simulink model "RealAndSimulatedPlantBlock2019"  (R2019b)
settings: Solver=FixedStepAuto  StartTime=0.0  StopTime=60  FixedStep=0.001  RelTol=1e-3
values from neighbouring files (symbols this model uses):
  A = [0 0 0 0 1 -7.46314951586 0 9.2203186001 0 -3.6743536316 0 36.5167723042 ... (16 elements, 4x4)]    [PlantParams.mat]
  B = [0 5.59662878796 0 -6.91433293703]    [PlantParams.mat]
  c = 0.2    [PlantParams.mat]    (also in params.m = 0.1)
  dtheta1 = 41.8879020479    [PlantParams.mat]    (also in params.m)
  g = 9.81    [PlantParams.mat]    (also in params.m)
  Id = 0.0148    [PlantParams.mat]    (also in params.m)
  ID = 0.0148142940058    [PlantParams.mat]
  J1 = 0.13138281053    [PlantParams.mat]    (also in params.m = 0.1314)
  JC = 0.0268600431258    [PlantParams.mat]
  JD = 0.0273039035837    [PlantParams.mat]
  Jz_bar = 0.0130765    [PlantParams.mat]    (also in params.m = 0.0131)
  lcg = 0.269778481013    [PlantParams.mat]    (also in params.m = 0.2698)
  m = 0.158    [PlantParams.mat]    (also in params.m)
  rh = 0.37    [PlantParams.mat]    (also in params.m)
undefined symbols (not defined in the file or in its folder): C, D, X, Y, Z
libraries: sm_lib x20, nesl_utility x5, simulink x1
(part 2 of 2)

== matlab function RealAndSimulatedPlantBlock2019/Plant/Non-linear Simulation Plant/Subsystem/MATLAB Function ==
  data: theta_ddot_1 output; theta_2 input; theta_3 input; theta_4 input; theta_dot_1 input; theta_dot_2 input; theta_dot_3 input; theta_dot_4 input; T_1 input; T_2 input; theta_ddot_2 output; theta_ddot_3 output; theta_ddot_4 output
function [theta_ddot_1, theta_ddot_2, theta_ddot_3, theta_ddot_4] = ...
    fcn(theta_2, theta_3, theta_4, theta_dot_1,...
        theta_dot_2, theta_dot_3, theta_dot_4, T_1, T_2)
g = 9.81;
theta_ddot_1 = -(1958372730237732701804682603107415175787744873616217473024000*T_1 - 366215700554455999080225274065048781396920318332014769625*theta_dot_1 + 237406127304858667686861471985309025571272801769849956875*theta_dot_1*cos(theta_2)^2 + 128809573249597331393363802079739755825647516562164812750*theta_dot_1*cos(theta_3)^2 + 217352965440431972313920503751859592659321613927317504000*theta_dot_1*cos(theta_4)^2 + 52359703185237910572295885124678117792802251079355468750*theta_dot_1*sin(theta_3)^2 + 3427789003866943481470413557670984804612355776241773576192*theta_dot_3*sin(theta_2) - 1269551482913682770914967984322586964671242880089545768960000*T_1*cos(theta_2)^2 - 688821247324049930889714618784828211116501993526671704064000*T_1*cos(theta_3)^2 - 1162315323210866213387287415560227994624885237945177473024000*T_1*cos(theta_4)^2 - 279998412755282956590263894637395024770552498749440000000000*T_1*sin(theta_3)^2 - 53471220207419015071532913264009106990133399900755204620000*theta_dot_2*theta_dot_3*cos(theta_2) + 753492488642099239087836691412794808278935743167945768960000*T_1*cos(theta_2)^2*cos(theta_4)^2 + 408822834568766974299450724147433186345949494777231704064000*T_1*cos(theta_3)^2*cos(theta_4)^2 - 140903095376072551492852586796797954626476348444508160000*theta_dot_1*cos(theta_2)^2*cos(theta_4)^2 - 76449870064359420821067916955061638032845265482809344000*theta_dot_1*cos(theta_3)^2*cos(theta_4)^2 + 9403754461680578526877673084778282939987100019066108660000*theta_dot_3^2*sin(2*theta_3)*sin(theta_2) + 34663711284057858017777567094452541110159199862622987300000*theta_dot_2*theta_dot_3*cos(theta_2)^3 - 516058994271583531827131292909792156392307136921600000000000*T_2*sin(theta_2)*sin(theta_3) + 6089496132404685675560149256335547445429224215674880000000*theta_dot_2*sin(theta_2)*sin(theta_3) + 688821247324049930889714618784828211116501993526671704064000*T_1*cos(theta_2)^2*cos(theta_3) - 128809573249597331393363802079739755825647516562164812750*theta_dot_1*cos(theta_2)^2*cos(theta_3) - 2034429719333667945537159066814545982353126506553453576192*theta_dot_3*cos(theta_4)^2*sin(theta_2) + 34663711284057858017777567094452541110159199862622987300000*theta_dot_1*theta_dot_2*cos(theta_2)*sin(theta_2) + 76449870064359420821067916955061638032845265482809344000*theta_dot_1*cos(theta_2)^2*cos(theta_3)*cos(theta_4)^2 - 9403754461680578526877673084778282939987100019066108660000*theta_dot_3^2*cos(theta_2)^2*sin(theta_2)*sin(theta_3) - 7045212511554242352783209429865101928420942356832031250000*theta_dot_3^2*sin(2*theta_2)*sin(theta_2)*sin(theta_3) + 18807508923361157053755346169556565879974200038132217320000*theta_dot_2*theta_dot_3*cos(theta_2)*cos(theta_3)^2 + 31735745518842579422338363526619723554514196982000517120000*theta_dot_2*theta_dot_3*cos(theta_2)*cos(theta_4)^2 - 18807508923361157053755346169556565879974200038132217320000*theta_dot_2*theta_dot_3*cos(theta_2)^3*cos(theta_3) + 7645049665467950943628130877659179578777318205090625000000*theta_dot_2*theta_dot_3*cos(theta_2)*sin(theta_3)^2 + 34663711284057858017777567094452541110159199862622987300000*theta_dot_2*theta_dot_3*sin(2*theta_2)*sin(theta_2) + 7077726405892498128003306834840222747846164275527680000*theta_dot_4*cos(theta_4)*sin(theta_2)*sin(theta_3) - 5581229628946603055063607645948693150598440916520796160000*theta_dot_3^2*sin(2*theta_3)*cos(theta_4)^2*sin(theta_2) - 20573286260949373312211148234722337253317315148958924800000*theta_dot_2*theta_dot_3*cos(theta_2)^3*cos(theta_4)^2 - 7645049665467950943628130877659179578777318205090625000000*theta_dot_3^2*cos(theta_3)*sin(theta_2)*sin(theta_3) + 8138895413405711776328644403303559546502173933174784000000*theta_dot_4^2*sin(theta_2)*sin(theta_3)*sin(theta_4) - 408822834568766974299450724147433186345949494777231704064000*T_1*cos(theta_2)^2*cos(theta_3)*cos(theta_4)^2 + 7645049665467950943628130877659179578777318205090625000000*theta_dot_3^2*cos(theta_2)*cos(theta_3)*sin(theta_2)^2*sin(theta_3) - 20573286260949373312211148234722337253317315148958924800000*theta_dot_1*theta_dot_2*cos(theta_2)*cos(theta_4)^2*sin(theta_2) - 37615017846722314107510692339113131759948400076264434640000*theta_dot_2*theta_dot_3*cos(theta_2)*cos(theta_3)*sin(theta_2)^2 - 30168808805116773270614095383506449462694275224436736000000*g*cos(theta_4)*sin(theta_2)*sin(theta_3)*sin(theta_4) + 5581229628946603055063607645948693150598440916520796160000*theta_dot_3^2*cos(theta_2)^2*cos(theta_4)^2*sin(theta_2)*sin(theta_3) - 11162459257893206110127215291897386301196881833041592320000*theta_dot_2*theta_dot_3*cos(theta_2)*cos(theta_3)^2*cos(theta_4)^2 + 11162459257893206110127215291897386301196881833041592320000*theta_dot_2*theta_dot_3*cos(theta_2)^3*cos(theta_3)*cos(theta_4)^2 - 20573286260949373312211148234722337253317315148958924800000*theta_dot_2*theta_dot_3*sin(2*theta_2)*cos(theta_4)^2*sin(theta_2) - 14090425023108484705566418859730203856841884713664062500000*theta_dot_1*theta_dot_3*cos(theta_2)*sin(theta_2)*sin(theta_3) + 22324918515786412220254430583794772602393763666083184640000*theta_dot_2*theta_dot_3*cos(theta_2)*cos(theta_3)*cos(theta_4)^2*sin(theta_2)^2)/(10734426842075824580000*(3229209327524243103578455495267868185*cos(theta_2)^2 + 1752073883408586258584044588908630554*cos(theta_3)^2 + 2956445275163430863787903017879076864*cos(theta_4)^2 + 3229209327524243103578455495267868185*sin(theta_2)^2 + 712199149329667464909054858375156250*sin(theta_3)^2 - 1752073883408586258584044588908630554*cos(theta_2)^2*cos(theta_3) - 1916570541084512070112913287345602560*cos(theta_2)^2*cos(theta_4)^2 - 1039874734078918793674989730533474304*cos(theta_3)^2*cos(theta_4)^2 - 1916570541084512070112913287345602560*cos(theta_4)^2*sin(theta_2)^2 + 1039874734078918793674989730533474304*cos(theta_2)^2*cos(theta_3)*cos(theta_4)^2 - 4981283210932829362162500084176498739));
theta_ddot_2 = (8799655665284731983770664469744582656000*theta_dot_2 - 7457335309563332189636156330292019200000000*T_2 - 5704540165669006975595484450903818240000*theta_dot_2*cos(theta_2)^2 - 3095115499615725008175180018840764416000*theta_dot_2*cos(theta_3)^2 - 110475157775578382071318015937187337500000*theta_dot_3^2*cos(theta_3) - 5704540165669006975595484450903818240000*theta_dot_2*sin(theta_2)^2 + 117611499500950702795799230524118007808000*theta_dot_4^2*sin(theta_4) + 38857585587426656885438033072948525000000*theta_dot_3^2*cos(theta_3)^3 - 101807182141934847986128970358377296875000*theta_dot_3^2*sin(2*theta_2) + 10227702573538355420671664494284374016*theta_dot_4*cos(theta_4) + 7082043939798692815316089873618698240000*theta_dot_3*sin(theta_3) + 4834356072600853369148715636359168000000000*T_2*cos(theta_2)^2 + 2622979236962478820487440693932851200000000*T_2*cos(theta_3)^2 + 4834356072600853369148715636359168000000000*T_2*sin(theta_2)^2 - 203614364283869695972257940716754593750000*theta_dot_1*theta_dot_3*cos(theta_2) + 71617572188151725185879982864238812500000*theta_dot_3^2*cos(theta_2)^2*cos(theta_3) + 71617572188151725185879982864238812500000*theta_dot_3^2*cos(theta_3)*sin(theta_2)^2 - 76243838210006208698186681479929528320000*theta_dot_4^2*cos(theta_2)^2*sin(theta_4) - 41367661290944494097612549044188479488000*theta_dot_4^2*cos(theta_3)^2*sin(theta_4) + 19428792793713328442719016536474262500000*theta_dot_3^2*sin(2*theta_3)*sin(theta_3) - 76243838210006208698186681479929528320000*theta_dot_4^2*sin(theta_2)^2*sin(theta_4) + 131996792095717970786377957852515781250000*theta_dot_1*theta_dot_3*cos(theta_2)^3 + 2622979236962478820487440693932851200000000*T_1*sin(theta_2)*sin(theta_3) - 435955822197072399806129699068871442432000*g*cos(theta_4)*sin(theta_4) - 38857585587426656885438033072948525000000*theta_dot_3^2*cos(theta_2)^2*cos(theta_3)^2 - 490497117311983517790668165856205859375*theta_dot_1*sin(theta_2)*sin(theta_3) + 65998396047858985393188978926257890625000*theta_dot_3^2*sin(2*theta_2)*cos(theta_2)^2 + 35808786094075862592939991432119406250000*theta_dot_3^2*sin(2*theta_2)*cos(theta_3)^2 - 19428792793713328442719016536474262500000*theta_dot_3^2*cos(theta_2)^2*sin(theta_3)^2 + 65998396047858985393188978926257890625000*theta_dot_3^2*sin(2*theta_2)*sin(theta_2)^2 - 2622979236962478820487440693932851200000000*T_2*cos(theta_2)^2*cos(theta_3) + 3095115499615725008175180018840764416000*theta_dot_2*cos(theta_2)^2*cos(theta_3) - 6630298088076149864174402723790192640*theta_dot_4*cos(theta_2)^2*cos(theta_4) - 3597404485462205556497261770494181376*theta_dot_4*cos(theta_3)^2*cos(theta_4) - 6630298088076149864174402723790192640*theta_dot_4*cos(theta_4)*sin(theta_2)^2 + 71617572188151725185879982864238812500000*theta_dot_1*theta_dot_2*cos(theta_2)*sin(theta_3) - 71617572188151725185879982864238812500000*theta_dot_3^2*cos(theta_2)*cos(theta_3)*sin(theta_2)^3 - 38857585587426656885438033072948525000000*theta_dot_3^2*cos(theta_2)*cos(theta_3)^3*sin(theta_2) - 71617572188151725185879982864238812500000*theta_dot_3^2*cos(theta_2)^3*cos(theta_3)*sin(theta_2) + 41367661290944494097612549044188479488000*theta_dot_4^2*cos(theta_2)^2*cos(theta_3)*sin(theta_4) + 71617572188151725185879982864238812500000*theta_dot_1*theta_dot_3*cos(theta_2)*cos(theta_3)^2 - 71617572188151725185879982864238812500000*theta_dot_1*theta_dot_3*cos(theta_2)^3*cos(theta_3) + 131996792095717970786377957852515781250000*theta_dot_1*theta_dot_3*cos(theta_2)*sin(theta_2)^2 + 71617572188151725185879982864238812500000*theta_dot_2*theta_dot_3*sin(2*theta_2)*sin(theta_3) - 35808786094075862592939991432119406250000*theta_dot_3^2*sin(2*theta_2)*cos(theta_2)^2*cos(theta_3) + 38857585587426656885438033072948525000000*theta_dot_3^2*cos(theta_2)^3*cos(theta_3)^2*sin(theta_2) + 3597404485462205556497261770494181376*theta_dot_4*cos(theta_2)^2*cos(theta_3)*cos(theta_4) + 282616456004245887960433916101556961280000*g*cos(theta_2)^2*cos(theta_4)*sin(theta_4) + 153339366192826511845695782967314481152000*g*cos(theta_3)^2*cos(theta_4)*sin(theta_4) + 110475157775578382071318015937187337500000*theta_dot_3^2*cos(theta_2)*cos(theta_3)*sin(theta_2) + 282616456004245887960433916101556961280000*g*cos(theta_4)*sin(theta_2)^2*sin(theta_4) - 153339366192826511845695782967314481152000*g*cos(theta_2)^2*cos(theta_3)*cos(theta_4)*sin(theta_4) - 71617572188151725185879982864238812500000*theta_dot_2*theta_dot_3*cos(theta_2)*sin(theta_2)*sin(theta_3) - 77715171174853313770876066145897050000000*theta_dot_2*theta_dot_3*cos(theta_2)*cos(theta_3)*sin(theta_2)*sin(theta_3))/(54560*(3229209327524243103578455495267868185*cos(theta_2)^2 + 1752073883408586258584044588908630554*cos(theta_3)^2 + 2956445275163430863787903017879076864*cos(theta_4)^2 + 3229209327524243103578455495267868185*sin(theta_2)^2 + 712199149329667464909054858375156250*sin(theta_3)^2 - 1752073883408586258584044588908630554*cos(theta_2)^2*cos(theta_3) - 1916570541084512070112913287345602560*cos(theta_2)^2*cos(theta_4)^2 - 1039874734078918793674989730533474304*cos(theta_3)^2*cos(theta_4)^2 - 1916570541084512070112913287345602560*cos(theta_4)^2*sin(theta_2)^2 + 1039874734078918793674989730533474304*cos(theta_2)^2*cos(theta_3)*cos(theta_4)^2 - 4981283210932829362162500084176498739));
theta_ddot_3 = -(1292552540529728278812357032543287580295168*theta_dot_3*cos(theta_4)^2 - 2177808033004564880726868266745624860295168*theta_dot_3 - 5974571942423279141771592048178430189140000*theta_dot_3^2*sin(2*theta_3) - 806595567779468474343284543239120318627840000*T_1*sin(theta_2) + 327872404620309852560930086741606400000000000*T_2*sin(theta_3) + 150833371174760598047502619515482357061875*theta_dot_1*sin(theta_2) - 3868894374519656260218975023550955520000000*theta_dot_2*sin(theta_3) - 5170957661368061762201568630523559936000000*theta_dot_4^2*sin(theta_3)*sin(theta_4) - 22023207613715337966405066477726861021700000*theta_dot_1*theta_dot_2*cos(theta_2) + 5974571942423279141771592048178430189140000*theta_dot_3^2*cos(theta_2)^2*sin(theta_3) + 4476098261759482824117498929014925781250000*theta_dot_3^2*sin(2*theta_2)*sin(theta_3) - 22023207613715337966405066477726861021700000*theta_dot_2*theta_dot_3*sin(2*theta_2) - 4496755606827756945621577213117726720000*theta_dot_4*cos(theta_4)*sin(theta_3) + 3545972843209113086431714981119147376640000*theta_dot_3^2*sin(2*theta_3)*cos(theta_4)^2 + 478723163159158621782354456497513918627840000*T_1*cos(theta_4)^2*sin(theta_2) - 89521231510762658323669098783456624640000*theta_dot_1*cos(theta_4)^2*sin(theta_2) + 4857198198428332110679754134118565625000000*theta_dot_3^2*cos(theta_3)*sin(theta_3) + 8952196523518965648234997858029851562500000*theta_dot_1*theta_dot_3*cos(theta_2)*sin(theta_3) + 22023207613715337966405066477726861021700000*theta_dot_2*theta_dot_3*cos(theta_2)*sin(theta_2) + 13071011090196372318170068619697009459200000*theta_dot_1*theta_dot_2*cos(theta_2)*cos(theta_4)^2 + 19167420774103313980711972870914310144000000*g*cos(theta_4)*sin(theta_3)*sin(theta_4) - 3545972843209113086431714981119147376640000*theta_dot_3^2*cos(theta_2)^2*cos(theta_4)^2*sin(theta_3) + 13071011090196372318170068619697009459200000*theta_dot_2*theta_dot_3*sin(2*theta_2)*cos(theta_4)^2 - 13071011090196372318170068619697009459200000*theta_dot_2*theta_dot_3*cos(theta_2)*cos(theta_4)^2*sin(theta_2) - 4857198198428332110679754134118565625000000*theta_dot_3^2*cos(theta_2)*cos(theta_3)*sin(theta_2)*sin(theta_3) + 23898287769693116567086368192713720756560000*theta_dot_2*theta_dot_3*cos(theta_2)*cos(theta_3)*sin(theta_2) - 14183891372836452345726859924476589506560000*theta_dot_2*theta_dot_3*cos(theta_2)*cos(theta_3)*cos(theta_4)^2*sin(theta_2))/(6820000*(3229209327524243103578455495267868185*cos(theta_2)^2 + 1752073883408586258584044588908630554*cos(theta_3)^2 + 2956445275163430863787903017879076864*cos(theta_4)^2 + 3229209327524243103578455495267868185*sin(theta_2)^2 + 712199149329667464909054858375156250*sin(theta_3)^2 - 1752073883408586258584044588908630554*cos(theta_2)^2*cos(theta_3) - 1916570541084512070112913287345602560*cos(theta_2)^2*cos(theta_4)^2 - 1039874734078918793674989730533474304*cos(theta_3)^2*cos(theta_4)^2 - 1916570541084512070112913287345602560*cos(theta_4)^2*sin(theta_2)^2 + 1039874734078918793674989730533474304*cos(theta_2)^2*cos(theta_3)*cos(theta_4)^2 - 4981283210932829362162500084176498739));
% theta_ddot_4 = (79*(1275208501998804316713600021549183677184*theta_dot_4 - 826677587846206234516084606788574255360*theta_dot_4*cos(theta_2)^2 - 448530914152598082197515414760609421824*theta_dot_4*cos(theta_3)^2 - 826677587846206234516084606788574255360*theta_dot_4*sin(theta_2)^2 - 182322982228394871016718043744040000000*theta_dot_4*sin(theta_3)^2 - 55184281290768658203307556844160942080000000*T_2*cos(theta_4) + 651174519231070166799029170761099116544000*theta_dot_2*cos(theta_4) - 5435576239769903399991720091853395423996800*g*sin(theta_4) + 287546133346957260952241444739819085000000*theta_dot_3^2*cos(theta_3)^3*cos(theta_4) - 753373147850317875097354380651991996875000*theta_dot_3^2*sin(2*theta_2)*cos(theta_4) + 52407125154510326833339065064778366976000*theta_dot_3*cos(theta_4)*sin(theta_3) + 35774234937246314931700495709057843200000000*T_2*cos(theta_2)^2*cos(theta_4) + 19410046353522343271607061135103098880000000*T_2*cos(theta_3)^2*cos(theta_4) + 35774234937246314931700495709057843200000000*T_2*cos(theta_4)*sin(theta_2)^2 - 422135972259506516194065849366882549760000*theta_dot_2*cos(theta_2)^2*cos(theta_4) - 229038546971563650604963321394216566784000*theta_dot_2*cos(theta_3)^2*cos(theta_4) + 448530914152598082197515414760609421824*theta_dot_4*cos(theta_2)^2*cos(theta_3) - 817516167539280027327753317935186297500000*theta_dot_3^2*cos(theta_3)*cos(theta_4) + 3523713218194454074624810636436297763472000*g*cos(theta_2)^2*sin(theta_4) + 1911863021575449325366909455417097660524800*g*cos(theta_3)^2*sin(theta_4) - 422135972259506516194065849366882549760000*theta_dot_2*cos(theta_4)*sin(theta_2)^2 + 870325096307035200688914305878473257779200*theta_dot_4^2*cos(theta_4)*sin(theta_4) + 3523713218194454074624810636436297763472000*g*sin(theta_2)^2*sin(theta_4) + 777151711748533137708760661458970500000000*g*sin(theta_3)^2*sin(theta_4) + 529970034192322766375511873195367212500000*theta_dot_3^2*cos(theta_2)^2*cos(theta_3)*cos(theta_4) + 529970034192322766375511873195367212500000*theta_dot_3^2*cos(theta_3)*cos(theta_4)*sin(theta_2)^2 - 564204402754045944366581442951478509568000*theta_dot_4^2*cos(theta_2)^2*cos(theta_4)*sin(theta_4) - 306120693552989256322332862926994748211200*theta_dot_4^2*cos(theta_3)^2*cos(theta_4)*sin(theta_4) + 143773066673478630476120722369909542500000*theta_dot_3^2*sin(2*theta_3)*cos(theta_4)*sin(theta_3) - 564204402754045944366581442951478509568000*theta_dot_4^2*cos(theta_4)*sin(theta_2)^2*sin(theta_4) + 976776261508312983819196888108616781250000*theta_dot_1*theta_dot_3*cos(theta_2)^3*cos(theta_4) + 19410046353522343271607061135103098880000000*T_1*cos(theta_4)*sin(theta_2)*sin(theta_3) - 287546133346957260952241444739819085000000*theta_dot_3^2*cos(theta_2)^2*cos(theta_3)^2*cos(theta_4) - 3629678668108678031650944427335923359375*theta_dot_1*cos(theta_4)*sin(theta_2)*sin(theta_3) + 488388130754156491909598444054308390625000*theta_dot_3^2*sin(2*theta_2)*cos(theta_2)^2*cos(theta_4) + 264985017096161383187755936597683606250000*theta_dot_3^2*sin(2*theta_2)*cos(theta_3)^2*cos(theta_4) - 143773066673478630476120722369909542500000*theta_dot_3^2*cos(theta_2)^2*cos(theta_4)*sin(theta_3)^2 + 488388130754156491909598444054308390625000*theta_dot_3^2*sin(2*theta_2)*cos(theta_4)*sin(theta_2)^2 - 19410046353522343271607061135103098880000000*T_2*cos(theta_2)^2*cos(theta_3)*cos(theta_4) + 229038546971563650604963321394216566784000*theta_dot_2*cos(theta_2)^2*cos(theta_3)*cos(theta_4) - 1911863021575449325366909455417097660524800*g*cos(theta_2)^2*cos(theta_3)*sin(theta_4) - 1506746295700635750194708761303983993750000*theta_dot_1*theta_dot_3*cos(theta_2)*cos(theta_4) - 529970034192322766375511873195367212500000*theta_dot_3^2*cos(theta_2)*cos(theta_3)*cos(theta_4)*sin(theta_2)^3 - 287546133346957260952241444739819085000000*theta_dot_3^2*cos(theta_2)*cos(theta_3)^3*cos(theta_4)*sin(theta_2) - 529970034192322766375511873195367212500000*theta_dot_3^2*cos(theta_2)^3*cos(theta_3)*cos(theta_4)*sin(theta_2) + 306120693552989256322332862926994748211200*theta_dot_4^2*cos(theta_2)^2*cos(theta_3)*cos(theta_4)*sin(theta_4) + 529970034192322766375511873195367212500000*theta_dot_1*theta_dot_3*cos(theta_2)*cos(theta_3)^2*cos(theta_4) - 529970034192322766375511873195367212500000*theta_dot_1*theta_dot_3*cos(theta_2)^3*cos(theta_3)*cos(theta_4) + 976776261508312983819196888108616781250000*theta_dot_1*theta_dot_3*cos(theta_2)*cos(theta_4)*sin(theta_2)^2 + 529970034192322766375511873195367212500000*theta_dot_2*theta_dot_3*sin(2*theta_2)*cos(theta_4)*sin(theta_3) - 264985017096161383187755936597683606250000*theta_dot_3^2*sin(2*theta_2)*cos(theta_2)^2*cos(theta_3)*cos(theta_4) + 287546133346957260952241444739819085000000*theta_dot_3^2*cos(theta_2)^3*cos(theta_3)^2*cos(theta_4)*sin(theta_2) + 817516167539280027327753317935186297500000*theta_dot_3^2*cos(theta_2)*cos(theta_3)*cos(theta_4)*sin(theta_2) + 529970034192322766375511873195367212500000*theta_dot_1*theta_dot_2*cos(theta_2)*cos(theta_4)*sin(theta_3) - 529970034192322766375511873195367212500000*theta_dot_2*theta_dot_3*cos(theta_2)*cos(theta_4)*sin(theta_2)*sin(theta_3) - 575092266693914521904482889479638170000000*theta_dot_2*theta_dot_3*cos(theta_2)*cos(theta_3)*cos(theta_4)*sin(theta_2)*sin(theta_3)))/(23256200*(3229209327524243103578455495267868185*cos(theta_2)^2 + 1752073883408586258584044588908630554*cos(theta_3)^2 + 2956445275163430863787903017879076864*cos(theta_4)^2 + 3229209327524243103578455495267868185*sin(theta_2)^2 + 712199149329667464909054858375156250*sin(theta_3)^2 - 1752073883408586258584044588908630554*cos(theta_2)^2*cos(theta_3) - 1916570541084512070112913287345602560*cos(theta_2)^2*cos(theta_4)^2 - 1039874734078918793674989730533474304*cos(theta_3)^2*cos(theta_4)^2 - 1916570541084512070112913287345602560*cos(theta_4)^2*sin(theta_2)^2 + 1039874734078918793674989730533474304*cos(theta_2)^2*cos(theta_3)*cos(theta_4)^2 - 4981283210932829362162500084176498739));
theta_ddot_4 = (79*(637604250999402158356800010774591838592*theta_dot_4 - 413338793923103117258042303394287127680*theta_dot_4*cos(theta_2)^2 - 224265457076299041098757707380304710912*theta_dot_4*cos(theta_3)^2 - 413338793923103117258042303394287127680*theta_dot_4*sin(theta_2)^2 - 91161491114197435508359021872020000000*theta_dot_4*sin(theta_3)^2 - 275921406453843291016537784220804710400000000*T_2*cos(theta_4) + 325587259615535083399514585380549558272000*theta_dot_2*cos(theta_4) - 27177881198849516999958600459266977119984000*g*sin(theta_4) + 1437730666734786304761207223699095425000000*theta_dot_3^2*cos(theta_3)^3*cos(theta_4) - 3766865739251589375486771903259959984375000*theta_dot_3^2*sin(2*theta_2)*cos(theta_4) + 262035625772551634166695325323891834880000*theta_dot_3*cos(theta_4)*sin(theta_3) + 178871174686231574658502478545289216000000000*T_2*cos(theta_2)^2*cos(theta_4) + 97050231767611716358035305675515494400000000*T_2*cos(theta_3)^2*cos(theta_4) + 178871174686231574658502478545289216000000000*T_2*cos(theta_4)*sin(theta_2)^2 - 211067986129753258097032924683441274880000*theta_dot_2*cos(theta_2)^2*cos(theta_4) - 114519273485781825302481660697108283392000*theta_dot_2*cos(theta_3)^2*cos(theta_4) + 224265457076299041098757707380304710912*theta_dot_4*cos(theta_2)^2*cos(theta_3) - 4087580837696400136638766589675931487500000*theta_dot_3^2*cos(theta_3)*cos(theta_4) + 17618566090972270373124053182181488817360000*g*cos(theta_2)^2*sin(theta_4) + 9559315107877246626834547277085488302624000*g*cos(theta_3)^2*sin(theta_4) - 211067986129753258097032924683441274880000*theta_dot_2*cos(theta_4)*sin(theta_2)^2 + 4351625481535176003444571529392366288896000*theta_dot_4^2*cos(theta_4)*sin(theta_4) + 17618566090972270373124053182181488817360000*g*sin(theta_2)^2*sin(theta_4) + 3885758558742665688543803307294852500000000*g*sin(theta_3)^2*sin(theta_4) + 2649850170961613831877559365976836062500000*theta_dot_3^2*cos(theta_2)^2*cos(theta_3)*cos(theta_4) + 2649850170961613831877559365976836062500000*theta_dot_3^2*cos(theta_3)*cos(theta_4)*sin(theta_2)^2 - 2821022013770229721832907214757392547840000*theta_dot_4^2*cos(theta_2)^2*cos(theta_4)*sin(theta_4) - 1530603467764946281611664314634973741056000*theta_dot_4^2*cos(theta_3)^2*cos(theta_4)*sin(theta_4) + 718865333367393152380603611849547712500000*theta_dot_3^2*sin(2*theta_3)*cos(theta_4)*sin(theta_3) - 2821022013770229721832907214757392547840000*theta_dot_4^2*cos(theta_4)*sin(theta_2)^2*sin(theta_4) + 4883881307541564919095984440543083906250000*theta_dot_1*theta_dot_3*cos(theta_2)^3*cos(theta_4) + 97050231767611716358035305675515494400000000*T_1*cos(theta_4)*sin(theta_2)*sin(theta_3) - 1437730666734786304761207223699095425000000*theta_dot_3^2*cos(theta_2)^2*cos(theta_3)^2*cos(theta_4) - 18148393340543390158254722136679616796875*theta_dot_1*cos(theta_4)*sin(theta_2)*sin(theta_3) + 2441940653770782459547992220271541953125000*theta_dot_3^2*sin(2*theta_2)*cos(theta_2)^2*cos(theta_4) + 1324925085480806915938779682988418031250000*theta_dot_3^2*sin(2*theta_2)*cos(theta_3)^2*cos(theta_4) - 718865333367393152380603611849547712500000*theta_dot_3^2*cos(theta_2)^2*cos(theta_4)*sin(theta_3)^2 + 2441940653770782459547992220271541953125000*theta_dot_3^2*sin(2*theta_2)*cos(theta_4)*sin(theta_2)^2 - 97050231767611716358035305675515494400000000*T_2*cos(theta_2)^2*cos(theta_3)*cos(theta_4) + 114519273485781825302481660697108283392000*theta_dot_2*cos(theta_2)^2*cos(theta_3)*cos(theta_4) - 9559315107877246626834547277085488302624000*g*cos(theta_2)^2*cos(theta_3)*sin(theta_4) - 7533731478503178750973543806519919968750000*theta_dot_1*theta_dot_3*cos(theta_2)*cos(theta_4) - 2649850170961613831877559365976836062500000*theta_dot_3^2*cos(theta_2)*cos(theta_3)*cos(theta_4)*sin(theta_2)^3 - 1437730666734786304761207223699095425000000*theta_dot_3^2*cos(theta_2)*cos(theta_3)^3*cos(theta_4)*sin(theta_2) - 2649850170961613831877559365976836062500000*theta_dot_3^2*cos(theta_2)^3*cos(theta_3)*cos(theta_4)*sin(theta_2) + 1530603467764946281611664314634973741056000*theta_dot_4^2*cos(theta_2)^2*cos(theta_3)*cos(theta_4)*sin(theta_4) + 2649850170961613831877559365976836062500000*theta_dot_1*theta_dot_3*cos(theta_2)*cos(theta_3)^2*cos(theta_4) - 2649850170961613831877559365976836062500000*theta_dot_1*theta_dot_3*cos(theta_2)^3*cos(theta_3)*cos(theta_4) + 4883881307541564919095984440543083906250000*theta_dot_1*theta_dot_3*cos(theta_2)*cos(theta_4)*sin(theta_2)^2 + 2649850170961613831877559365976836062500000*theta_dot_2*theta_dot_3*sin(2*theta_2)*cos(theta_4)*sin(theta_3) - 1324925085480806915938779682988418031250000*theta_dot_3^2*sin(2*theta_2)*cos(theta_2)^2*cos(theta_3)*cos(theta_4) + 1437730666734786304761207223699095425000000*theta_dot_3^2*cos(theta_2)^3*cos(theta_3)^2*cos(theta_4)*sin(theta_2) + 4087580837696400136638766589675931487500000*theta_dot_3^2*cos(theta_2)*cos(theta_3)*cos(theta_4)*sin(theta_2) + 2649850170961613831877559365976836062500000*theta_dot_1*theta_dot_2*cos(theta_2)*cos(theta_4)*sin(theta_3) - 2649850170961613831877559365976836062500000*theta_dot_2*theta_dot_3*cos(theta_2)*cos(theta_4)*sin(theta_2)*sin(theta_3) - 2875461333469572609522414447398190850000000*theta_dot_2*theta_dot_3*cos(theta_2)*cos(theta_3)*cos(theta_4)*sin(theta_2)*sin(theta_3)))/(116281000*(3229209327524243103578455495267868185*cos(theta_2)^2 + 1752073883408586258584044588908630554*cos(theta_3)^2 + 2956445275163430863787903017879076864*cos(theta_4)^2 + 3229209327524243103578455495267868185*sin(theta_2)^2 + 712199149329667464909054858375156250*sin(theta_3)^2 - 1752073883408586258584044588908630554*cos(theta_2)^2*cos(theta_3) - 1916570541084512070112913287345602560*cos(theta_2)^2*cos(theta_4)^2 - 1039874734078918793674989730533474304*cos(theta_3)^2*cos(theta_4)^2 - 1916570541084512070112913287345602560*cos(theta_4)^2*sin(theta_2)^2 + 1039874734078918793674989730533474304*cos(theta_2)^2*cos(theta_3)*cos(theta_4)^2 - 4981283210932829362162500084176498739));
end
